simulink model "ECS787"  (R2013a)
settings: Solver=ode45  StartTime=0.0  StopTime=10000  RelTol=1e-3
InitFcn:
  | load('SampleOutput.mat')
  | 
  | load('SampleFuelBurn.mat')
undefined symbols (not defined in the file): AirProp
libraries: PowerFlowLib x8, simulink x4
(part 6 of 6)

== system ECS787/Left Pack/Primary HX (air-air)/HX_and_Fin_paramters/HX_parameters/Calculating the no of passages per fluid flow ==
  Raw_HX_parameters : Inport
  Fin_parameters : Inport  Port=2
  Add : Sum  Inputs=+---
  Add1 : Sum  Inputs=+++
  Bus Selector : BusSelector  OutputSignals=H_hx,t_p
  Bus Selector1 : BusSelector  OutputSignals=h_fin,t_fin
  Display : Display
  Divide : Product  Inputs=*/
  Gain{,1..3} (4 alike) : Gain  Gain=2
  Rounding Function : Rounding  Operator=round
  N_passages_per_flow : Outport
  wires:
  Rounding Function/1 -> Display/1, N_passages_per_flow/1
  Divide/1 -> Rounding Function/1
  Add1/1 -> Divide/2
  Add/1 -> Divide/1
  Gain3/1 -> Add1/3
  Gain2/1 -> Add1/2
  Gain1/1 -> Add1/1
  Gain/1 -> Add/4
  Bus Selector/2 -> Gain3/1, Gain/1  "<t_p>"
  Bus Selector1/2 -> Gain2/1, Add/3  "<t_fin>"
  Bus Selector1/1 -> Gain1/1, Add/2  "<h_fin>"
  Bus Selector/1 -> Add/1  "<H_hx>"
  Fin_parameters/1 -> Bus Selector1/1
  Raw_HX_parameters/1 -> Bus Selector/1

== system ECS787/Left Pack/Primary HX (air-air)/HX_and_Fin_paramters/HX_parameters/Calculating the total number of fins per HX per fluid flow ==
  Raw_HX_parameters : Inport
  Fin_parameters : Inport  Port=2
  N_passages_per_flow : Inport  Port=3
  Bus Selector : BusSelector  OutputSignals=W_hx,L_hx
  Bus Selector1 : BusSelector  OutputSignals=s_fin,t_fin,l_fin
  Divide : Product  Inputs=***//
  Rounding Function : Rounding  Operator=round
  s+t : Sum
  Tot_no_of_fins_per_HX_per_flow : Outport
  wires:
  Rounding Function/1 -> Tot_no_of_fins_per_HX_per_flow/1
  Divide/1 -> Rounding Function/1
  Bus Selector1/3 -> Divide/5  "<l_fin>"
  s+t/1 -> Divide/4  "s+t"
  N_passages_per_flow/1 -> Divide/3
  Bus Selector/2 -> Divide/2  "<L_hx>"
  Bus Selector/1 -> Divide/1  "<W_hx>"
  Bus Selector1/2 -> s+t/2  "<t_fin>"
  Bus Selector1/1 -> s+t/1  "<s_fin>"
  Fin_parameters/1 -> Bus Selector1/1
  Raw_HX_parameters/1 -> Bus Selector/1

== system ECS787/Left Pack/Primary HX (air-air)/HX_and_Fin_paramters/HX_parameters/Calculating total free flow area per flow ==
  Raw_HX_parameters : Inport
  Fin_parameters : Inport  Port=2
  N_passages_per_flow : Inport  Port=3
  "Calculating the per fin ratio of the free flow area to the frontal area " : Subsystem
  Calculating total passages area per flow : Subsystem
  Product : Product  RndMeth=Zero
  Total_free_flow_area : Outport
  wires:
  Product/1 -> Total_free_flow_area/1
  Calculating total passages area per flow/1(total_pasages_area_per_flow) -> Product/2
  "Calculating the per fin ratio of the free flow area to the frontal area "/1(Per fin ratio of the free flow to the frontal areas) -> Product/1
  N_passages_per_flow/1 -> Calculating total passages area per flow/3(N_passages_per_flow)
  Raw_HX_parameters/1 -> Calculating total passages area per flow/2("HX_parameters ")
  Fin_parameters/1 -> Calculating total passages area per flow/1(Fin_parameters), "Calculating the per fin ratio of the free flow area to the frontal area "/1(Fin_parameters)

== system ECS787/Left Pack/Secondary HX (air-air)1/HX_and_Fin_paramters/HX_parameters/Calculating the no of passages per fluid flow ==
  Raw_HX_parameters : Inport
  Fin_parameters : Inport  Port=2
  Add : Sum  Inputs=+---
  Add1 : Sum  Inputs=+++
  Bus Selector : BusSelector  OutputSignals=H_hx,t_p
  Bus Selector1 : BusSelector  OutputSignals=h_fin,t_fin
  Display : Display
  Divide : Product  Inputs=*/
  Gain{,1..3} (4 alike) : Gain  Gain=2
  Rounding Function : Rounding  Operator=round
  N_passages_per_flow : Outport
  wires:
  Rounding Function/1 -> Display/1, N_passages_per_flow/1
  Divide/1 -> Rounding Function/1
  Add1/1 -> Divide/2
  Add/1 -> Divide/1
  Gain3/1 -> Add1/3
  Gain2/1 -> Add1/2
  Gain1/1 -> Add1/1
  Gain/1 -> Add/4
  Bus Selector/2 -> Gain3/1, Gain/1  "<t_p>"
  Bus Selector1/2 -> Gain2/1, Add/3  "<t_fin>"
  Bus Selector1/1 -> Gain1/1, Add/2  "<h_fin>"
  Bus Selector/1 -> Add/1  "<H_hx>"
  Fin_parameters/1 -> Bus Selector1/1
  Raw_HX_parameters/1 -> Bus Selector/1

== system ECS787/Left Pack/Secondary HX (air-air)1/HX_and_Fin_paramters/HX_parameters/Calculating the total number of fins per HX per fluid flow ==
  Raw_HX_parameters : Inport
  Fin_parameters : Inport  Port=2
  N_passages_per_flow : Inport  Port=3
  Bus Selector : BusSelector  OutputSignals=W_hx,L_hx
  Bus Selector1 : BusSelector  OutputSignals=s_fin,t_fin,l_fin
  Divide : Product  Inputs=***//
  Rounding Function : Rounding  Operator=round
  s+t : Sum
  Tot_no_of_fins_per_HX_per_flow : Outport
  wires:
  Rounding Function/1 -> Tot_no_of_fins_per_HX_per_flow/1
  Divide/1 -> Rounding Function/1
  Bus Selector1/3 -> Divide/5  "<l_fin>"
  s+t/1 -> Divide/4  "s+t"
  N_passages_per_flow/1 -> Divide/3
  Bus Selector/2 -> Divide/2  "<L_hx>"
  Bus Selector/1 -> Divide/1  "<W_hx>"
  Bus Selector1/2 -> s+t/2  "<t_fin>"
  Bus Selector1/1 -> s+t/1  "<s_fin>"
  Fin_parameters/1 -> Bus Selector1/1
  Raw_HX_parameters/1 -> Bus Selector/1

== system ECS787/Left Pack/Secondary HX (air-air)1/HX_and_Fin_paramters/HX_parameters/Calculating total free flow area per flow ==
  Raw_HX_parameters : Inport
  Fin_parameters : Inport  Port=2
  N_passages_per_flow : Inport  Port=3
  "Calculating the per fin ratio of the free flow area to the frontal area " : Subsystem
  Calculating total passages area per flow : Subsystem
  Product : Product  RndMeth=Zero
  Total_free_flow_area : Outport
  wires:
  Product/1 -> Total_free_flow_area/1
  Calculating total passages area per flow/1(total_pasages_area_per_flow) -> Product/2
  "Calculating the per fin ratio of the free flow area to the frontal area "/1(Per fin ratio of the free flow to the frontal areas) -> Product/1
  N_passages_per_flow/1 -> Calculating total passages area per flow/3(N_passages_per_flow)
  Raw_HX_parameters/1 -> Calculating total passages area per flow/2("HX_parameters ")
  Fin_parameters/1 -> Calculating total passages area per flow/1(Fin_parameters), "Calculating the per fin ratio of the free flow area to the frontal area "/1(Fin_parameters)

== system ECS787/Right Pack1/Primary HX (air-air)/HX_and_Fin_paramters/HX_parameters/Calculating the no of passages per fluid flow ==
  Raw_HX_parameters : Inport
  Fin_parameters : Inport  Port=2
  Add : Sum  Inputs=+---
  Add1 : Sum  Inputs=+++
  Bus Selector : BusSelector  OutputSignals=H_hx,t_p
  Bus Selector1 : BusSelector  OutputSignals=h_fin,t_fin
  Display : Display
  Divide : Product  Inputs=*/
  Gain{,1..3} (4 alike) : Gain  Gain=2
  Rounding Function : Rounding  Operator=round
  N_passages_per_flow : Outport
  wires:
  Rounding Function/1 -> Display/1, N_passages_per_flow/1
  Divide/1 -> Rounding Function/1
  Add1/1 -> Divide/2
  Add/1 -> Divide/1
  Gain3/1 -> Add1/3
  Gain2/1 -> Add1/2
  Gain1/1 -> Add1/1
  Gain/1 -> Add/4
  Bus Selector/2 -> Gain3/1, Gain/1  "<t_p>"
  Bus Selector1/2 -> Gain2/1, Add/3  "<t_fin>"
  Bus Selector1/1 -> Gain1/1, Add/2  "<h_fin>"
  Bus Selector/1 -> Add/1  "<H_hx>"
  Fin_parameters/1 -> Bus Selector1/1
  Raw_HX_parameters/1 -> Bus Selector/1

== system ECS787/Right Pack1/Primary HX (air-air)/HX_and_Fin_paramters/HX_parameters/Calculating the total number of fins per HX per fluid flow ==
  Raw_HX_parameters : Inport
  Fin_parameters : Inport  Port=2
  N_passages_per_flow : Inport  Port=3
  Bus Selector : BusSelector  OutputSignals=W_hx,L_hx
  Bus Selector1 : BusSelector  OutputSignals=s_fin,t_fin,l_fin
  Divide : Product  Inputs=***//
  Rounding Function : Rounding  Operator=round
  s+t : Sum
  Tot_no_of_fins_per_HX_per_flow : Outport
  wires:
  Rounding Function/1 -> Tot_no_of_fins_per_HX_per_flow/1
  Divide/1 -> Rounding Function/1
  Bus Selector1/3 -> Divide/5  "<l_fin>"
  s+t/1 -> Divide/4  "s+t"
  N_passages_per_flow/1 -> Divide/3
  Bus Selector/2 -> Divide/2  "<L_hx>"
  Bus Selector/1 -> Divide/1  "<W_hx>"
  Bus Selector1/2 -> s+t/2  "<t_fin>"
  Bus Selector1/1 -> s+t/1  "<s_fin>"
  Fin_parameters/1 -> Bus Selector1/1
  Raw_HX_parameters/1 -> Bus Selector/1

== system ECS787/Right Pack1/Primary HX (air-air)/HX_and_Fin_paramters/HX_parameters/Calculating total free flow area per flow ==
  Raw_HX_parameters : Inport
  Fin_parameters : Inport  Port=2
  N_passages_per_flow : Inport  Port=3
  "Calculating the per fin ratio of the free flow area to the frontal area " : Subsystem
  Calculating total passages area per flow : Subsystem
  Product : Product  RndMeth=Zero
  Total_free_flow_area : Outport
  wires:
  Product/1 -> Total_free_flow_area/1
  Calculating total passages area per flow/1(total_pasages_area_per_flow) -> Product/2
  "Calculating the per fin ratio of the free flow area to the frontal area "/1(Per fin ratio of the free flow to the frontal areas) -> Product/1
  N_passages_per_flow/1 -> Calculating total passages area per flow/3(N_passages_per_flow)
  Raw_HX_parameters/1 -> Calculating total passages area per flow/2("HX_parameters ")
  Fin_parameters/1 -> Calculating total passages area per flow/1(Fin_parameters), "Calculating the per fin ratio of the free flow area to the frontal area "/1(Fin_parameters)

== system ECS787/Right Pack1/Secondary HX (air-air)1/HX_and_Fin_paramters/HX_parameters/Calculating the no of passages per fluid flow ==
  Raw_HX_parameters : Inport
  Fin_parameters : Inport  Port=2
  Add : Sum  Inputs=+---
  Add1 : Sum  Inputs=+++
  Bus Selector : BusSelector  OutputSignals=H_hx,t_p
  Bus Selector1 : BusSelector  OutputSignals=h_fin,t_fin
  Display : Display
  Divide : Product  Inputs=*/
  Gain{,1..3} (4 alike) : Gain  Gain=2
  Rounding Function : Rounding  Operator=round
  N_passages_per_flow : Outport
  wires:
  Rounding Function/1 -> Display/1, N_passages_per_flow/1
  Divide/1 -> Rounding Function/1
  Add1/1 -> Divide/2
  Add/1 -> Divide/1
  Gain3/1 -> Add1/3
  Gain2/1 -> Add1/2
  Gain1/1 -> Add1/1
  Gain/1 -> Add/4
  Bus Selector/2 -> Gain3/1, Gain/1  "<t_p>"
  Bus Selector1/2 -> Gain2/1, Add/3  "<t_fin>"
  Bus Selector1/1 -> Gain1/1, Add/2  "<h_fin>"
  Bus Selector/1 -> Add/1  "<H_hx>"
  Fin_parameters/1 -> Bus Selector1/1
  Raw_HX_parameters/1 -> Bus Selector/1

== system ECS787/Right Pack1/Secondary HX (air-air)1/HX_and_Fin_paramters/HX_parameters/Calculating the total number of fins per HX per fluid flow ==
  Raw_HX_parameters : Inport
  Fin_parameters : Inport  Port=2
  N_passages_per_flow : Inport  Port=3
  Bus Selector : BusSelector  OutputSignals=W_hx,L_hx
  Bus Selector1 : BusSelector  OutputSignals=s_fin,t_fin,l_fin
  Divide : Product  Inputs=***//
  Rounding Function : Rounding  Operator=round
  s+t : Sum
  Tot_no_of_fins_per_HX_per_flow : Outport
  wires:
  Rounding Function/1 -> Tot_no_of_fins_per_HX_per_flow/1
  Divide/1 -> Rounding Function/1
  Bus Selector1/3 -> Divide/5  "<l_fin>"
  s+t/1 -> Divide/4  "s+t"
  N_passages_per_flow/1 -> Divide/3
  Bus Selector/2 -> Divide/2  "<L_hx>"
  Bus Selector/1 -> Divide/1  "<W_hx>"
  Bus Selector1/2 -> s+t/2  "<t_fin>"
  Bus Selector1/1 -> s+t/1  "<s_fin>"
  Fin_parameters/1 -> Bus Selector1/1
  Raw_HX_parameters/1 -> Bus Selector/1

== system ECS787/Right Pack1/Secondary HX (air-air)1/HX_and_Fin_paramters/HX_parameters/Calculating total free flow area per flow ==
  Raw_HX_parameters : Inport
  Fin_parameters : Inport  Port=2
  N_passages_per_flow : Inport  Port=3
  "Calculating the per fin ratio of the free flow area to the frontal area " : Subsystem
  Calculating total passages area per flow : Subsystem
  Product : Product  RndMeth=Zero
  Total_free_flow_area : Outport
  wires:
  Product/1 -> Total_free_flow_area/1
  Calculating total passages area per flow/1(total_pasages_area_per_flow) -> Product/2
  "Calculating the per fin ratio of the free flow area to the frontal area "/1(Per fin ratio of the free flow to the frontal areas) -> Product/1
  N_passages_per_flow/1 -> Calculating total passages area per flow/3(N_passages_per_flow)
  Raw_HX_parameters/1 -> Calculating total passages area per flow/2("HX_parameters ")
  Fin_parameters/1 -> Calculating total passages area per flow/1(Fin_parameters), "Calculating the per fin ratio of the free flow area to the frontal area "/1(Fin_parameters)

== system ECS787/Left Pack/Primary HX (air-air)/HX_and_Fin_paramters/HX_parameters/Calculating total free flow area per flow/Calculating the per fin ratio of the free flow area to the frontal area  ==
  Fin_parameters : Inport
  Bus Selector1 : BusSelector  OutputSignals=s_fin,t_fin,h_fin
  Divide : Product  Inputs=**//
  h+t : Sum
  s+t : Sum
  s-t : Sum  Inputs=+-
  Per fin ratio of the free flow to the frontal areas : Outport
  wires:
  Divide/1 -> Per fin ratio of the free flow to the frontal areas/1
  h+t/1 -> Divide/4  "h+t"
  s+t/1 -> Divide/3  "s+t"
  s-t/1 -> Divide/1  "s-t"
  Bus Selector1/3 -> Divide/2, h+t/2  "<h_fin>"
  Bus Selector1/2 -> h+t/1, s+t/2, s-t/2  "<t_fin>"
  Bus Selector1/1 -> s+t/1, s-t/1  "<s_fin>"
  Fin_parameters/1 -> Bus Selector1/1

== system ECS787/Left Pack/Primary HX (air-air)/HX_and_Fin_paramters/HX_parameters/Calculating total free flow area per flow/Calculating total passages area per flow ==
  Fin_parameters : Inport
  "HX_parameters " : Inport  Port=2
  N_passages_per_flow : Inport  Port=3
  Bus Selector : BusSelector  OutputSignals=h_fin,t_fin
  Bus Selector1 : BusSelector  OutputSignals=W_hx
  Divide : Product  Inputs=***
  h+t : Sum
  total_pasages_area_per_flow : Outport
  wires:
  Divide/1 -> total_pasages_area_per_flow/1
  Bus Selector1/1 -> Divide/2  "<W_hx>"
  h+t/1 -> Divide/1
  Bus Selector/2 -> h+t/2  "<t_fin>"
  Bus Selector/1 -> h+t/1  "<h_fin>"
  N_passages_per_flow/1 -> Divide/3
  "HX_parameters "/1 -> Bus Selector1/1
  Fin_parameters/1 -> Bus Selector/1

== system ECS787/Left Pack/Secondary HX (air-air)1/HX_and_Fin_paramters/HX_parameters/Calculating total free flow area per flow/Calculating the per fin ratio of the free flow area to the frontal area  ==
  Fin_parameters : Inport
  Bus Selector1 : BusSelector  OutputSignals=s_fin,t_fin,h_fin
  Divide : Product  Inputs=**//
  h+t : Sum
  s+t : Sum
  s-t : Sum  Inputs=+-
  Per fin ratio of the free flow to the frontal areas : Outport
  wires:
  Divide/1 -> Per fin ratio of the free flow to the frontal areas/1
  h+t/1 -> Divide/4  "h+t"
  s+t/1 -> Divide/3  "s+t"
  s-t/1 -> Divide/1  "s-t"
  Bus Selector1/3 -> Divide/2, h+t/2  "<h_fin>"
  Bus Selector1/2 -> h+t/1, s+t/2, s-t/2  "<t_fin>"
  Bus Selector1/1 -> s+t/1, s-t/1  "<s_fin>"
  Fin_parameters/1 -> Bus Selector1/1

== system ECS787/Left Pack/Secondary HX (air-air)1/HX_and_Fin_paramters/HX_parameters/Calculating total free flow area per flow/Calculating total passages area per flow ==
  Fin_parameters : Inport
  "HX_parameters " : Inport  Port=2
  N_passages_per_flow : Inport  Port=3
  Bus Selector : BusSelector  OutputSignals=h_fin,t_fin
  Bus Selector1 : BusSelector  OutputSignals=W_hx
  Divide : Product  Inputs=***
  h+t : Sum
  total_pasages_area_per_flow : Outport
  wires:
  Divide/1 -> total_pasages_area_per_flow/1
  Bus Selector1/1 -> Divide/2  "<W_hx>"
  h+t/1 -> Divide/1
  Bus Selector/2 -> h+t/2  "<t_fin>"
  Bus Selector/1 -> h+t/1  "<h_fin>"
  N_passages_per_flow/1 -> Divide/3
  "HX_parameters "/1 -> Bus Selector1/1
  Fin_parameters/1 -> Bus Selector/1

== system ECS787/Right Pack1/Primary HX (air-air)/HX_and_Fin_paramters/HX_parameters/Calculating total free flow area per flow/Calculating the per fin ratio of the free flow area to the frontal area  ==
  Fin_parameters : Inport
  Bus Selector1 : BusSelector  OutputSignals=s_fin,t_fin,h_fin
  Divide : Product  Inputs=**//
  h+t : Sum
  s+t : Sum
  s-t : Sum  Inputs=+-
  Per fin ratio of the free flow to the frontal areas : Outport
  wires:
  Divide/1 -> Per fin ratio of the free flow to the frontal areas/1
  h+t/1 -> Divide/4  "h+t"
  s+t/1 -> Divide/3  "s+t"
  s-t/1 -> Divide/1  "s-t"
  Bus Selector1/3 -> Divide/2, h+t/2  "<h_fin>"
  Bus Selector1/2 -> h+t/1, s+t/2, s-t/2  "<t_fin>"
  Bus Selector1/1 -> s+t/1, s-t/1  "<s_fin>"
  Fin_parameters/1 -> Bus Selector1/1

== system ECS787/Right Pack1/Primary HX (air-air)/HX_and_Fin_paramters/HX_parameters/Calculating total free flow area per flow/Calculating total passages area per flow ==
  Fin_parameters : Inport
  "HX_parameters " : Inport  Port=2
  N_passages_per_flow : Inport  Port=3
  Bus Selector : BusSelector  OutputSignals=h_fin,t_fin
  Bus Selector1 : BusSelector  OutputSignals=W_hx
  Divide : Product  Inputs=***
  h+t : Sum
  total_pasages_area_per_flow : Outport
  wires:
  Divide/1 -> total_pasages_area_per_flow/1
  Bus Selector1/1 -> Divide/2  "<W_hx>"
  h+t/1 -> Divide/1
  Bus Selector/2 -> h+t/2  "<t_fin>"
  Bus Selector/1 -> h+t/1  "<h_fin>"
  N_passages_per_flow/1 -> Divide/3
  "HX_parameters "/1 -> Bus Selector1/1
  Fin_parameters/1 -> Bus Selector/1

== system ECS787/Right Pack1/Secondary HX (air-air)1/HX_and_Fin_paramters/HX_parameters/Calculating total free flow area per flow/Calculating the per fin ratio of the free flow area to the frontal area  ==
  Fin_parameters : Inport
  Bus Selector1 : BusSelector  OutputSignals=s_fin,t_fin,h_fin
  Divide : Product  Inputs=**//
  h+t : Sum
  s+t : Sum
  s-t : Sum  Inputs=+-
  Per fin ratio of the free flow to the frontal areas : Outport
  wires:
  Divide/1 -> Per fin ratio of the free flow to the frontal areas/1
  h+t/1 -> Divide/4  "h+t"
  s+t/1 -> Divide/3  "s+t"
  s-t/1 -> Divide/1  "s-t"
  Bus Selector1/3 -> Divide/2, h+t/2  "<h_fin>"
  Bus Selector1/2 -> h+t/1, s+t/2, s-t/2  "<t_fin>"
  Bus Selector1/1 -> s+t/1, s-t/1  "<s_fin>"
  Fin_parameters/1 -> Bus Selector1/1

== system ECS787/Right Pack1/Secondary HX (air-air)1/HX_and_Fin_paramters/HX_parameters/Calculating total free flow area per flow/Calculating total passages area per flow ==
  Fin_parameters : Inport
  "HX_parameters " : Inport  Port=2
  N_passages_per_flow : Inport  Port=3
  Bus Selector : BusSelector  OutputSignals=h_fin,t_fin
  Bus Selector1 : BusSelector  OutputSignals=W_hx
  Divide : Product  Inputs=***
  h+t : Sum
  total_pasages_area_per_flow : Outport
  wires:
  Divide/1 -> total_pasages_area_per_flow/1
  Bus Selector1/1 -> Divide/2  "<W_hx>"
  h+t/1 -> Divide/1
  Bus Selector/2 -> h+t/2  "<t_fin>"
  Bus Selector/1 -> h+t/1  "<h_fin>"
  N_passages_per_flow/1 -> Divide/3
  "HX_parameters "/1 -> Bus Selector1/1
  Fin_parameters/1 -> Bus Selector/1
